simulink model "Car_State_ETR07_2"  (R2017b)
settings: Solver=VariableStepAuto  StartTime=0.0  StopTime=10.0  RelTol=1e-3
libraries: simulink x4
settings Model: Creator=cspt  LastModifiedBy=cspt

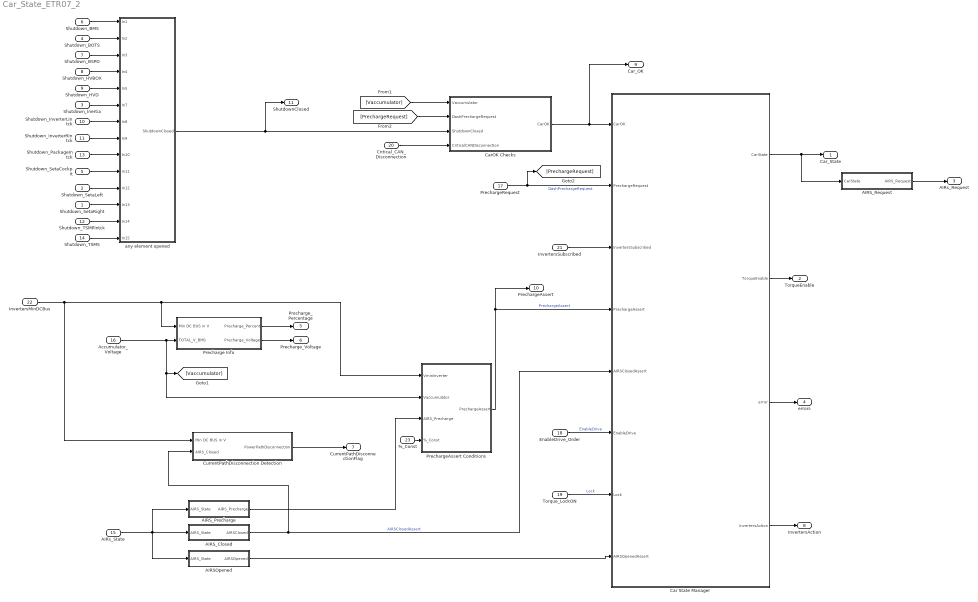
== system Car_State_ETR07_2 ==
  Shutdown_SetaRight : Inport
  Shutdown_SetaLeft : Inport  Port=2
  Shutdown_Inertia : Inport  Port=3
  Shutdown_BOTS : Inport  Port=4
  Shutdown_SetaCockpit : Inport  Port=5
  Shutdown_BMS : Inport  Port=6
  Shutdown_BSPD : Inport  Port=7
  Shutdown_HVBOX : Inport  Port=8
  Shutdown_HVD : Inport  Port=9
  Shutdown_InverterLIntck : Inport  Port=10
  Shutdown_InverterRIntck : Inport  Port=11
  Shutdown_TSMPIntck : Inport  Port=12
  Shutdown_PackageIntck : Inport  Port=13
  Shutdown_TSMS : Inport  Port=14
  AIRs_State : Inport  Port=15
  Accumulator_Voltage : Inport  Port=16
  PrechargeRequest : Inport  Port=17
  EnableDrive_Order : Inport  Port=18
  Torque_LockON : Inport  Port=19
  Critical_CAN_Disconnection : Inport  Port=20
  InvertersSubscribed : Inport  Port=21
  InvertersMinDCBus : Inport  Port=22
  %_Const : Inport  Port=23
  AIRSOpened : Subsystem
  AIRS_Closed : Subsystem
  AIRS_Precharge : Subsystem
  AIRS_Request : Subsystem
  Car State Manager : Stateflow chart  TreatAsAtomicUnit=on  SystemSampleTime=0.025
  CarOK Checks : Subsystem
  CurrentPathDisconnection Detection : Subsystem
  Precharge Info : Subsystem
  PrechargeAssert Conditions : Subsystem
  any element opened : Subsystem
  Car_State : Outport
  TorqueEnable : Outport  Port=2
  AIRs_Request : Outport  Port=3
  errors : Outport  Port=4
  Precharge_Percentage : Outport  Port=5
  Precharge_Voltage : Outport  Port=6
  CurrentPathDisconnectionFlag : Outport  Port=7
  InvertersAction : Outport  Port=8
  Car_OK : Outport  Port=9
  PrechargeAssert : Outport  Port=10
  ShutdownClosed : Outport  Port=11
  wires:
  AIRs_State/1 -> AIRSOpened/1(AIRS_State), AIRS_Precharge/1(AIRS_State), AIRS_Closed/1(AIRS_State)
  Car State Manager/3(error) -> errors/1
  EnableDrive_Order/1 -> Car State Manager/6(EnableDrive)  "EnableDrive"
  Shutdown_InverterRIntck/1 -> any element opened/8(In9)
  AIRSOpened/1(AIRSOpened) -> Car State Manager/8(AIRSOpenedAssert)
  any element opened/1(ShutdownClosed) -> ShutdownClosed/1, CarOK Checks/3(ShutdownClosed)
  Shutdown_BSPD/1 -> any element opened/3(In3)
  Accumulator_Voltage/1 -> PrechargeAssert Conditions/2(Vaccumulator), [Vaccumulator], Precharge Info/2(TOTAL_V_BMS)
  Precharge Info/2(Precharge_Voltage) -> Precharge_Voltage/1
  PrechargeRequest/1 -> [PrechargeRequest], Car State Manager/2(PrechargeRequest)  "DashPrechargeRequest"
  Torque_LockON/1 -> Car State Manager/7(Lock)  "Lock"
  PrechargeAssert Conditions/1(PrechargeAssert) -> PrechargeAssert/1, Car State Manager/4(PrechargeAssert)  "PrechargeAssert"
  CarOK Checks/1(CarOK) -> Car_OK/1, Car State Manager/1(CarOK)
  Car State Manager/4(InvertersAction) -> InvertersAction/1
  Shutdown_SetaCockpit/1 -> any element opened/10(In11)
  AIRS_Precharge/1(AIRS_Precharge) -> PrechargeAssert Conditions/3(AIRS_Precharge)
  Car State Manager/1(CarState) -> Car_State/1, AIRS_Request/1(CarState)
  Shutdown_PackageIntck/1 -> any element opened/9(In10)
  InvertersSubscribed/1 -> Car State Manager/3(InvertersSubscribed)
  Critical_CAN_Disconnection/1 -> CarOK Checks/4(CriticalCANDisconnection)
  Shutdown_Inertia/1 -> any element opened/6(In7)
  AIRS_Request/1(AIRS_Request) -> AIRs_Request/1
  [Vaccumulator] -> CarOK Checks/1(Vaccumulator)
  Shutdown_TSMS/1 -> any element opened/14(In15)
  Car State Manager/2(TorqueEnable) -> TorqueEnable/1
  Precharge Info/1(Precharge_Percent) -> Precharge_Percentage/1
  [PrechargeRequest] -> CarOK Checks/2(DashPrechargeRequest)
  Shutdown_BOTS/1 -> any element opened/2(In2)
  Shutdown_HVBOX/1 -> any element opened/4(In4)
  CurrentPathDisconnection Detection/1(PowerPathDisconnection) -> CurrentPathDisconnectionFlag/1
  Shutdown_InverterLIntck/1 -> any element opened/7(In8)
  Shutdown_HVD/1 -> any element opened/5(In5)
  AIRS_Closed/1(AIRSClosed) -> Car State Manager/5(AIRSClosedAssert), CurrentPathDisconnection Detection/2(AIRS_Closed)  "AIRSClosedAssert"
  Shutdown_BMS/1 -> any element opened/1(In1)
  Shutdown_SetaRight/1 -> any element opened/12(In13)
  InvertersMinDCBus/1 -> PrechargeAssert Conditions/1(VminInverter), Precharge Info/1(Min DC BUS in V), CurrentPathDisconnection Detection/1(Min DC BUS in V)
  Shutdown_TSMPIntck/1 -> any element opened/13(In14)
  Shutdown_SetaLeft/1 -> any element opened/11(In12)
  %_Const/1 -> PrechargeAssert Conditions/4(%_Const)

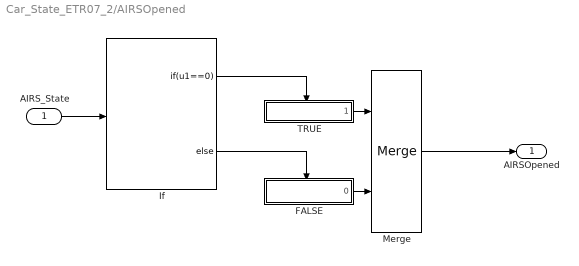
== system Car_State_ETR07_2/AIRSOpened ==
  AIRS_State : Inport
  FALSE : Subsystem  TreatAsAtomicUnit=on
  If : If  IfExpression=u1==0
  Merge : Merge
  TRUE : Subsystem  TreatAsAtomicUnit=on
  AIRSOpened : Outport
  wires:
  Merge/1 -> AIRSOpened/1
  FALSE/1(0) -> Merge/2
  If/2 -> FALSE/Action
  TRUE/1(1) -> Merge/1
  If/1 -> TRUE/Action
  AIRS_State/1 -> If/1

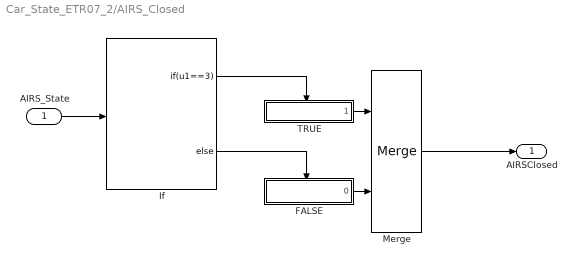
== system Car_State_ETR07_2/AIRS_Closed ==
  AIRS_State : Inport
  FALSE : Subsystem  TreatAsAtomicUnit=on
  If : If  IfExpression=u1==3
  Merge : Merge
  TRUE : Subsystem  TreatAsAtomicUnit=on
  AIRSClosed : Outport
  wires:
  Merge/1 -> AIRSClosed/1
  FALSE/1(0) -> Merge/2
  If/2 -> FALSE/Action
  TRUE/1(1) -> Merge/1
  If/1 -> TRUE/Action
  AIRS_State/1 -> If/1

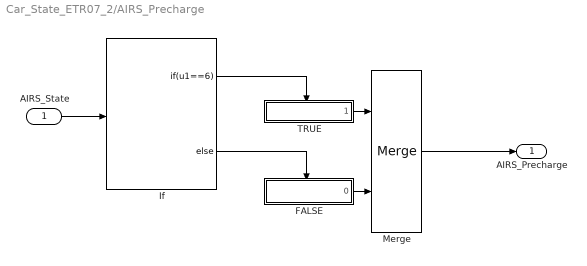
== system Car_State_ETR07_2/AIRS_Precharge ==
  AIRS_State : Inport
  FALSE : Subsystem  TreatAsAtomicUnit=on
  If : If  IfExpression=u1==6
  Merge : Merge
  TRUE : Subsystem  TreatAsAtomicUnit=on
  AIRS_Precharge : Outport
  wires:
  Merge/1 -> AIRS_Precharge/1
  FALSE/1(0) -> Merge/2
  If/2 -> FALSE/Action
  TRUE/1(1) -> Merge/1
  If/1 -> TRUE/Action
  AIRS_State/1 -> If/1

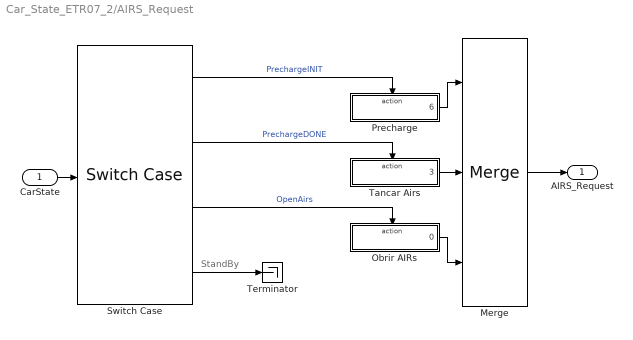
== system Car_State_ETR07_2/AIRS_Request ==
  note: StandBy
  CarState : Inport
  Merge : Merge  Inputs=3
  Obrir AIRs : Subsystem  TreatAsAtomicUnit=on
  Precharge : Subsystem  TreatAsAtomicUnit=on
  Switch Case : SwitchCase  CaseConditions={6,9,21}
  Tancar Airs : Subsystem  TreatAsAtomicUnit=on
  Terminator : Terminator
  AIRS_Request : Outport
  wires:
  Merge/1 -> AIRS_Request/1
  Switch Case/2 -> Tancar Airs/Action  "PrechargeDONE"
  Switch Case/1 -> Precharge/Action  "PrechargeINIT"
  CarState/1 -> Switch Case/1
  Switch Case/3 -> Obrir AIRs/Action  "OpenAirs"
  Precharge/1(6) -> Merge/1
  Tancar Airs/1(3) -> Merge/2
  Obrir AIRs/1(0) -> Merge/3
  Switch Case/4 -> Terminator/1

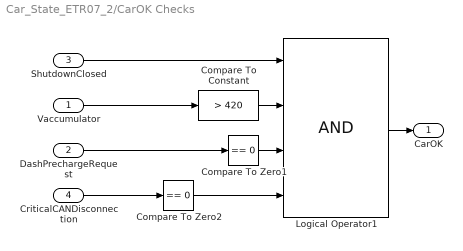
== system Car_State_ETR07_2/CarOK Checks ==
  Vaccumulator : Inport
  DashPrechargeRequest : Inport  Port=2
  ShutdownClosed : Inport  Port=3
  CriticalCANDisconnection : Inport  Port=4
  Compare To Constant : simulink/Logic and Bit Operations/Compare To Constant  relop=>  const=420  OutDataTypeStr=boolean
  Compare To Zero1 : simulink/Logic and Bit Operations/Compare To Zero  relop===  OutDataTypeStr=boolean
  Compare To Zero2 : simulink/Logic and Bit Operations/Compare To Zero  relop===  OutDataTypeStr=boolean
  Logical Operator1 : Logic  Inputs=4  AllPortsSameDT=off  OutDataTypeStr=boolean
  CarOK : Outport
  wires:
  ShutdownClosed/1 -> Logical Operator1/1
  Compare To Constant/1 -> Logical Operator1/2
  Logical Operator1/1 -> CarOK/1
  Vaccumulator/1 -> Compare To Constant/1
  DashPrechargeRequest/1 -> Compare To Zero1/1
  Compare To Zero1/1 -> Logical Operator1/3
  CriticalCANDisconnection/1 -> Compare To Zero2/1
  Compare To Zero2/1 -> Logical Operator1/4

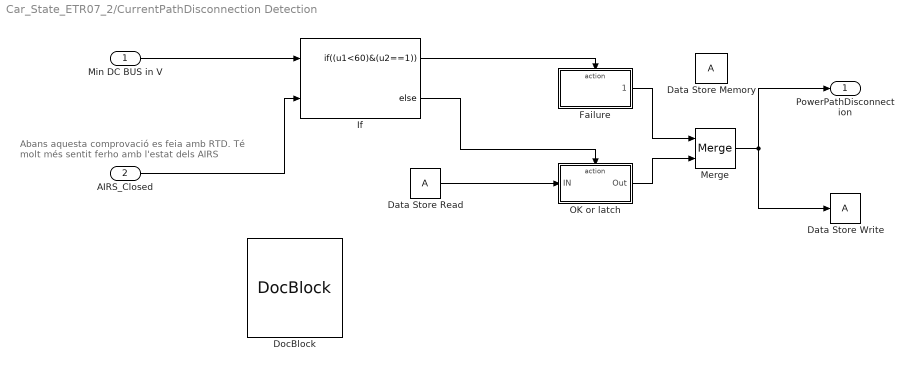
== system Car_State_ETR07_2/CurrentPathDisconnection Detection ==
  note: Abans aquesta comprovació es feia amb RTD.
      | Té molt més sentit ferho amb l'estat dels AIRS
  Min DC BUS in V : Inport
  AIRS_Closed : Inport  Port=2
  Data Store Memory : DataStoreMemory  ReadBeforeWriteMsg=warning  WriteAfterWriteMsg=warning  WriteAfterReadMsg=warning  ShowAdditionalParam=off
  Data Store Read : DataStoreRead
  Data Store Write : DataStoreWrite
  DocBlock : simulink/Model-Wide Utilities/DocBlock  DocumentType=Text
      content=|
      | This module checks if the power path is disconnected somehow.
      |
      | Examples of why this could happen:
      | - HVD Removed
      | - Blown Fuse
      | - Disconnected Cable
      | ...
  Failure : Subsystem  TreatAsAtomicUnit=on
  If : If  NumInputs=2  IfExpression=(u1<60)&(u2==1)
  Merge : Merge
  OK or latch : Subsystem  TreatAsAtomicUnit=on
  PowerPathDisconnection : Outport
  wires:
  OK or latch/1("Out ") -> Merge/2
  Merge/1 -> PowerPathDisconnection/1, Data Store Write/1
  If/2 -> OK or latch/Action
  Data Store Read/1 -> OK or latch/1(IN)
  If/1 -> Failure/Action
  Failure/1("1 ") -> Merge/1
  AIRS_Closed/1 -> If/2
  Min DC BUS in V/1 -> If/1

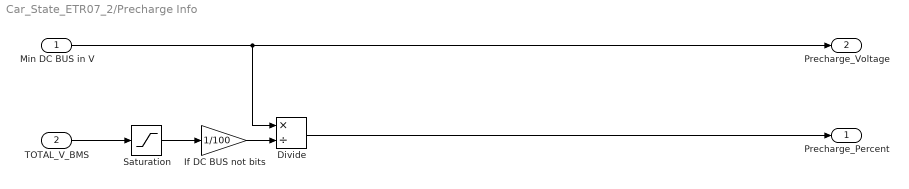
== system Car_State_ETR07_2/Precharge Info ==
  Min DC BUS in V : Inport
  TOTAL_V_BMS : Inport  Port=2
  Divide : Product  Inputs=*/
  If DC BUS not bits : Gain  Gain=1/100
  Saturation : Saturate  UpperLimit=600  LowerLimit=400
  Precharge_Percent : Outport
  Precharge_Voltage : Outport  Port=2
  wires:
  Divide/1 -> Precharge_Percent/1
  Saturation/1 -> If DC BUS not bits/1
  Min DC BUS in V/1 -> Precharge_Voltage/1, Divide/1
  TOTAL_V_BMS/1 -> Saturation/1
  If DC BUS not bits/1 -> Divide/2

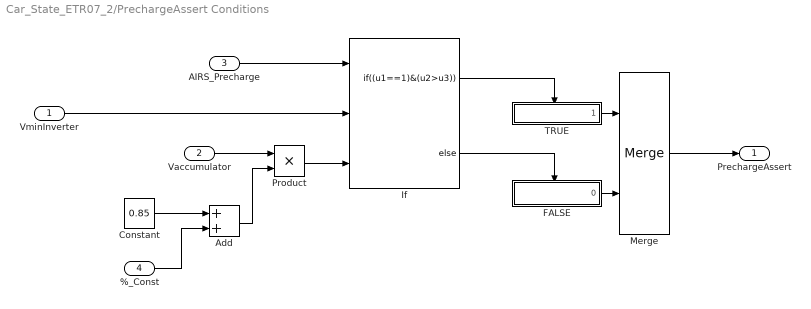
== system Car_State_ETR07_2/PrechargeAssert Conditions ==
  VminInverter : Inport
  Vaccumulator : Inport  Port=2
  AIRS_Precharge : Inport  Port=3
  %_Const : Inport  Port=4
  Add : Sum
  Constant : Constant  Value=0.85
  FALSE : Subsystem  TreatAsAtomicUnit=on
  If : If  NumInputs=3  IfExpression=(u1==1)&(u2>u3)
  Merge : Merge
  Product : Product
  TRUE : Subsystem  TreatAsAtomicUnit=on
  PrechargeAssert : Outport
  wires:
  Vaccumulator/1 -> Product/1
  If/2 -> FALSE/Action
  Product/1 -> If/3
  FALSE/1(0) -> Merge/2
  TRUE/1(1) -> Merge/1
  If/1 -> TRUE/Action
  Merge/1 -> PrechargeAssert/1
  VminInverter/1 -> If/2
  AIRS_Precharge/1 -> If/1
  Add/1 -> Product/2
  Constant/1 -> Add/1
  %_Const/1 -> Add/2

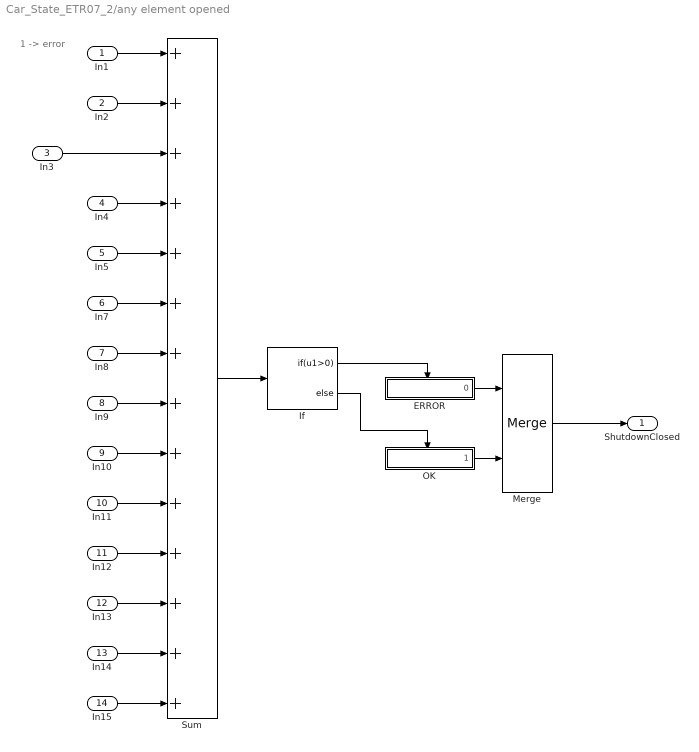
== system Car_State_ETR07_2/any element opened ==
  note: 1 -> error
  In1 : Inport
  In2 : Inport  Port=2
  In3 : Inport  Port=3
  In4 : Inport  Port=4
  In5 : Inport  Port=5
  In7 : Inport  Port=6
  In8 : Inport  Port=7
  In9 : Inport  Port=8
  In10 : Inport  Port=9
  In11 : Inport  Port=10
  In12 : Inport  Port=11
  In13 : Inport  Port=12
  In14 : Inport  Port=13
  In15 : Inport  Port=14
  ERROR : Subsystem  TreatAsAtomicUnit=on
  If : If  IfExpression=u1>0
  Merge : Merge
  OK : Subsystem  TreatAsAtomicUnit=on
  Sum : Sum  Inputs=++++++++++++++
  ShutdownClosed : Outport
  wires:
  In7/1 -> Sum/6
  In9/1 -> Sum/8
  In8/1 -> Sum/7
  In4/1 -> Sum/4
  In2/1 -> Sum/2
  In11/1 -> Sum/10
  In5/1 -> Sum/5
  Sum/1 -> If/1
  In1/1 -> Sum/1
  In12/1 -> Sum/11
  In10/1 -> Sum/9
  Merge/1 -> ShutdownClosed/1
  In13/1 -> Sum/12
  OK/1(1) -> Merge/2
  ERROR/1(0) -> Merge/1
  If/2 -> OK/Action
  If/1 -> ERROR/Action
  In14/1 -> Sum/13
  In15/1 -> Sum/14
  In3/1 -> Sum/3

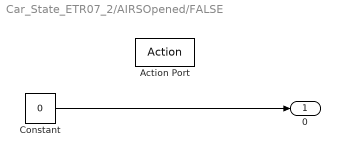
== system Car_State_ETR07_2/AIRSOpened/FALSE ==
  Action Port : ActionPort
  Constant : Constant  Value=0
  0 : Outport
  wires:
  Constant/1 -> 0/1

== system Car_State_ETR07_2/AIRSOpened/TRUE ==
  Action Port : ActionPort
  Constant : Constant
  1 : Outport
  wires:
  Constant/1 -> 1/1

== system Car_State_ETR07_2/AIRS_Closed/FALSE ==
  Action Port : ActionPort
  Constant : Constant  Value=0
  0 : Outport
  wires:
  Constant/1 -> 0/1

== system Car_State_ETR07_2/AIRS_Closed/TRUE ==
  Action Port : ActionPort
  Constant : Constant
  1 : Outport
  wires:
  Constant/1 -> 1/1

== system Car_State_ETR07_2/AIRS_Precharge/FALSE ==
  Action Port : ActionPort
  Constant : Constant  Value=0
  0 : Outport
  wires:
  Constant/1 -> 0/1

== system Car_State_ETR07_2/AIRS_Precharge/TRUE ==
  Action Port : ActionPort
  Constant : Constant
  1 : Outport
  wires:
  Constant/1 -> 1/1

== system Car_State_ETR07_2/AIRS_Request/Obrir AIRs ==
  Action Port : ActionPort
  Constant : Constant  Value=0
  0 : Outport
  wires:
  Constant/1 -> 0/1

== system Car_State_ETR07_2/AIRS_Request/Precharge ==
  Action Port : ActionPort
  Constant : Constant  Value=6
  6 : Outport
  wires:
  Constant/1 -> 6/1

== system Car_State_ETR07_2/AIRS_Request/Tancar Airs ==
  Action Port : ActionPort
  Constant : Constant  Value=3
  3 : Outport
  wires:
  Constant/1 -> 3/1

== system Car_State_ETR07_2/CurrentPathDisconnection Detection/Failure ==
  Action Port : ActionPort
  Constant : Constant
  "1 " : Outport
  wires:
  Constant/1 -> "1 "/1

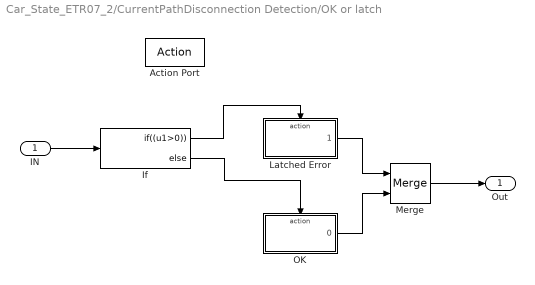
== system Car_State_ETR07_2/CurrentPathDisconnection Detection/OK or latch ==
  IN : Inport
  Action Port : ActionPort
  If : If  IfExpression=(u1>0)
  Latched Error : Subsystem  TreatAsAtomicUnit=on
  Merge : Merge
  OK : Subsystem  TreatAsAtomicUnit=on
  "Out " : Outport
  wires:
  IN/1 -> If/1
  If/1 -> Latched Error/Action
  If/2 -> OK/Action
  Latched Error/1("1 ") -> Merge/1
  OK/1("0 ") -> Merge/2
  Merge/1 -> "Out "/1

== system Car_State_ETR07_2/PrechargeAssert Conditions/FALSE ==
  Action Port : ActionPort
  Constant : Constant  Value=0
  0 : Outport
  wires:
  Constant/1 -> 0/1

== system Car_State_ETR07_2/PrechargeAssert Conditions/TRUE ==
  Action Port : ActionPort
  Constant : Constant
  1 : Outport
  wires:
  Constant/1 -> 1/1

== system Car_State_ETR07_2/any element opened/ERROR ==
  Action Port : ActionPort
  Constant : Constant  Value=0
  0 : Outport
  wires:
  Constant/1 -> 0/1

== system Car_State_ETR07_2/any element opened/OK ==
  Action Port : ActionPort
  Constant : Constant
  1 : Outport
  wires:
  Constant/1 -> 1/1

== system Car_State_ETR07_2/CurrentPathDisconnection Detection/OK or latch/Latched Error ==
  Action Port : ActionPort
  Constant : Constant
  "1 " : Outport
  wires:
  Constant/1 -> "1 "/1

== system Car_State_ETR07_2/CurrentPathDisconnection Detection/OK or latch/OK ==
  Action Port : ActionPort
  Constant : Constant  Value=0
  "0 " : Outport
  wires:
  Constant/1 -> "0 "/1

== stateflow chart Car_State_ETR07_2/Car State Manager ==
  state SAFESTATE [group]
    state Init
      entry: CarState=0;
      TorqueEnable=0;
      InvertersAction=20;
    state Standby
      entry: CarState=3;
      TorqueEnable=0;
      InvertersAction=11;
    (default) -> Init : {error=0}
    Standby -> Init [order 2] : [CarOK==0]
    Init -> Standby : [CarOK==1 & after(1, sec)]
  state STOP [group]
    state OpenAirs
      entry: CarState=21;
      InvertersAction=20;
  note: Inverter Actions that can be commanded to the inverters:
      |
      | Unsubscribe -> 10
      | Subscribe -> 11
      | DisableDrive -> 20
      | EnableDrive -> 21
      | TorqueCommand -> 30
  state PRECHARGE [group]
    state PrechargeINIT
      entry: CarState=6;
      TorqueEnable=0;
      InvertersAction=20;
    state PrechargeDONE
      entry: CarState=9;
      TorqueEnable=0;
      InvertersAction=20;
    PrechargeINIT -> PrechargeDONE [order 1] : [PrechargeAssert==1 & after(2500,msec)]
  state ACTIVE [group]
    state TSActive
      entry: CarState=12;
      TorqueEnable=0;
      InvertersAction=20;
    state EnableInverters
      entry: CarState=14;
      TorqueEnable=0;
      InvertersAction=21;
    state RTD
      entry: CarState=15;
      TorqueEnable=1;
      InvertersAction=30;
    state Locked
      entry: CarState=18;
      TorqueEnable=0;
      InvertersAction=20;
    RTD -> Locked [order 1] : [Lock==1]
    EnableInverters -> RTD [order 1] : [after(2,sec)]
    TSActive -> EnableInverters [order 1] : [EnableDrive==1]
    Locked -> EnableInverters [order 1] : [Lock==0]
  OpenAirs -> Init : [AIRSOpenedAssert==1 & after(1,sec)]
  Standby -> PrechargeINIT [order 1] : [PrechargeRequest==1 & InvertersSubscribed==1]
  PrechargeINIT -> OpenAirs [order 2] : after(10,sec)
      | {error=6}
  PrechargeDONE -> OpenAirs [order 1] : after(2,sec)
      | {error=9}
  TSActive -> OpenAirs [order 2] : [CarOK==0]
  EnableInverters -> OpenAirs [order 2] : [CarOK==0]
  RTD -> OpenAirs [order 2] : [CarOK==0]
  Locked -> OpenAirs [order 2] : [CarOK==0]
  PrechargeDONE -> TSActive [order 2] : [AIRSClosedAssert==1 & after(100,msec)]
  data: CarOK input; PrechargeRequest input; InvertersSubscribed input; CarState output double; PrechargeAssert input; AIRSClosedAssert input; EnableDrive input; Lock input double; AIRSOpenedAssert input; TorqueEnable output double; error output double; InvertersAction output double
